simulink model "persistent_params"  (Simulink 3.00)
undefined symbols (not defined in the file): ycn
libraries: mathlib x8, paramlib x4, execlib x2, logiclib x1, genlib x1, arclib x1

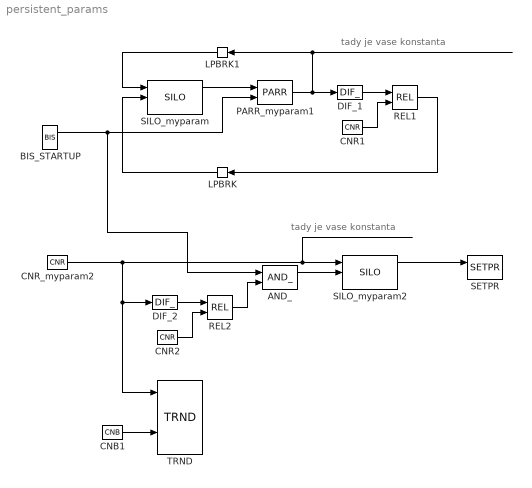
== system persistent_params ==
  note: tady je vase konstanta
  note: tady je vase konstanta
  AND_ : logiclib/AND_
  BIS_STARTUP : genlib/BIS  Y0=off  t1=1  t2=0  t3=3  t4=4  t5=5  t6=6  t7=7  t8=8  RPT=off
  CNB1 : mathlib/CNB  YCN=on
  CNR1 : mathlib/CNR  ycn=0
  CNR2 : mathlib/CNR  ycn=0
  CNR_myparam2 : mathlib/CNR  ycn=2
  DIF_1 : mathlib/DIF_
  DIF_2 : mathlib/DIF_
  LPBRK : execlib/LPBRK  Orientation=left
  LPBRK1 : execlib/LPBRK  Orientation=left
  PARR_myparam1 : paramlib/PARR  par=1  SATF=off  hilim=1  lolim=-1
  REL1 : mathlib/REL  irel=2: inequality (!=)
  REL2 : mathlib/REL  irel=2: inequality (!=)
  SETPR : paramlib/SETPR  sc=.CNR_myparam2:ycn  SETF=off
  SILO_myparam : paramlib/SILO  fname=myparam1.txt  CSF=off  CLF=off  yerr=0
  SILO_myparam2 : paramlib/SILO  fname=myparam2.txt  CSF=off  CLF=off  yerr=0
  TRND : arclib/TRND  n=1  l=10000  btype=8: Double  ptype1=1: Store  ptype2=1: Store  ptype3=1: Store  ptype4=1: Store  pfac=1  afac=0  arc=0  id=1  Title=Trend Title
  wires:
  AND_/1 -> SILO_myparam2/2
  BIS_STARTUP/1 -> AND_/1, PARR_myparam1/2
  CNB1/1 -> TRND/5
  CNR_myparam2/1 -> DIF_2/1, TRND/1, SILO_myparam2/1
  CNR1/1 -> REL1/2
  CNR2/1 -> REL2/2
  DIF_1/1 -> REL1/1
  DIF_2/1 -> REL2/1
  LPBRK/1 -> SILO_myparam/2
  LPBRK1/1 -> SILO_myparam/1
  PARR_myparam1/1 -> DIF_1/1, LPBRK1/1
  REL1/1 -> LPBRK/1
  REL2/1 -> AND_/2
  SILO_myparam/1 -> PARR_myparam1/1
  SILO_myparam2/1 -> SETPR/1
